simulink model "rlAutoParkingValet3D"  (R2024b)
settings: Solver=VariableStepAuto  StartTime=0.0  StopTime=inf  RelTol=1e-3  AbsTol=1e-4
InitFcn:
  | if ~doTraining
  |     setupActorVehicles(mdl,freeSpotIndex);
  | end
  | egoTargetPose = parkingLot.findGoalPose(vehiclePose,freeSpotIndex,searchDist);
StartFcn:
  | if exist("visualizer","var") && ~doTraining
  |     visualizer.resetVehicle(egoInitialPose,freeSpotIndex,doTraining);
  | end
model workspace: external: MAT-File (data not in the file)
values from neighbouring files (symbols this model uses):
  centerToRear = 1.343    [autoParkingValetParams3D.m]
  doTraining = false    [RL_Parking_And_Control.m]    (also in analisis.m; lanzarSimParalelas.m)
  egoInitialPose = [40 -55 pi/2]    [RL_Parking_And_Control.m]    (also in lanzarSimParalelas.m)
  freeSpotIndex = spotsToSimulate(i)    [RL_Parking_And_Control.m]    (also in analisis.m = 18; autoParkingValetResetFcn3D.m = 21; lanzarSimParalelas.m = 18)
  info = ParkingLotManager.getInfo()    [ParkingLotManager.m]    (also in ParkingLotVisualizer.m = this.Info; RL_Parking_And_Control.m = parkingLot.getInfo(); analisis.m = parkingLot.getInfo(); autoParkingValetResetFcn3D.m)
  K_lqr = dlqr(Ad, Bd, Q, R)    [createLQRForParking3D.m]
  maxLidarDist = 20    [autoParkingValetParams3D.m]
  parkingLot = obj.ParkingLot    [ModeSelector.m]    (also in RL_Parking_And_Control.m = ParkingLotManager; analisis.m = ParkingLotManager; lanzarSimParalelas.m = ParkingLotManager)
  pTracking = 10    [createMPCForParking3D.m]    (also in createNonLinearMPCForParking3D.m)
  searchDist = 10    [RL_Parking_And_Control.m]    (also in analisis.m; lanzarSimParalelas.m)
  speedMax = 2    [autoParkingValetParams3D.m]
  steerMax = pi/4    (= 0.785398163397)    [autoParkingValetParams3D.m]
  terrTol = deg2rad(10)    [autoParkingValetParams3D.m]
  Tf = 50    [RL_Parking_And_Control.m]    (also in analisis.m; lanzarSimParalelas.m)
  trainXBounds = info.TrainingZoneXLimits    [autoParkingValetParams3D.m]    (also in autoParkingValetResetFcn3D.m = [(info.SpotLocations(freeSpotIndex,1) - 6.8125)             )
  trainYBounds = info.TrainingZoneYLimits    [autoParkingValetParams3D.m]    (also in autoParkingValetResetFcn3D.m = [(info.SpotLocations(freeSpotIndex,2) - 9.56)              ()
  Ts = 0.1    [RL_Parking_And_Control.m]    (also in analisis.m; createMPCForParking3D.m; lanzarSimParalelas.m)
  vehiclePose = [10 -32.5 pi]    [RL_Parking_And_Control.m]    (also in analisis.m; lanzarSimParalelas.m)
  xBounds = info.XLimits    [autoParkingValetParams3D.m]
  Xref = [xRef(1:p,:);repmat(xRef(end,:),Tsteps-p,1)]    [ParkingLotManager.m]    (also in createLQRForParking3D.m = parkingLot.createReferenceTrajectory(Ts, Tf); createMPCForParking3D.m = ParkingLotManager.createReferenceTrajectory(Ts,Tf); createNonLinearMPCForParking3D.m = ParkingLotManager.createReferenceTrajectory(Ts,Tf))
  xyerrTol = 0.75    [autoParkingValetParams3D.m]
  yBounds = info.YLimits    [autoParkingValetParams3D.m]
undefined symbols (not defined in the file or in its folder): Sim3dSensor
libraries: sim3dautolib x23, simulink_extras x23, mpclib x2, rllib x1, robotmobilelib x1, sim3dphyssensorlib x1, sim3dlib x1
(part 2 of 2)

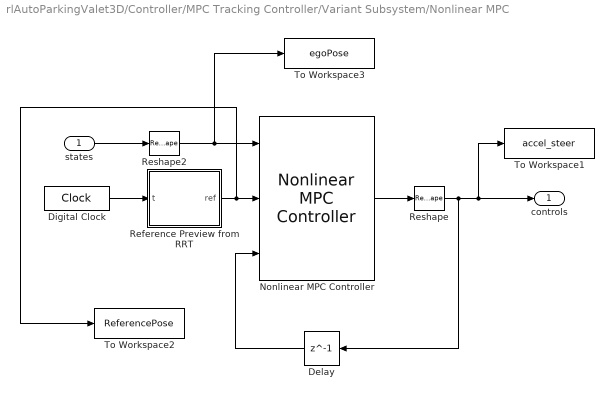
== system rlAutoParkingValet3D/Controller/MPC Tracking Controller/Variant Subsystem/Nonlinear MPC ==
  states : Inport
  Delay : Delay  DelayLength=1
  Digital Clock : DigitalClock  SampleTime=Ts
  Nonlinear MPC Controller : mpclib/Nonlinear MPC Controller  SCDEnableBlockLinearizationSpecification=on  nlmpcobj=nlobjTracking  UseObjectTs=on  UseMEX=off  md_enabled=off  mvtarget_enabled=off  param_enabled=off  cost_enabled=off  mvseq_enabled=off  stateseq_enabled=off  ovseq_enabled=off  slack_enabled=off  status_enabled=off  ov_min=off  ov_max=off  mv_min=off  mv_max=off  mvrate_min=off  mvrate_max=off  state_min=off  state_max=off  ov_weight=off  mv_weight=off  mvrate_weight=off  ecr_weight=off  nlp_initialize=off
  Reference Preview from RRT : MATLAB Function  TreatAsAtomicUnit=on
  Reshape : Reshape  OutputDimensionality=Customize  OutputDimensions=[2,1]
  Reshape2 : Reshape  OutputDimensionality=Customize  OutputDimensions=[3,1]
  To Workspace1 : ToWorkspace  VariableName=accel_steer  SaveFormat=Timeseries  SampleTime=-1
  To Workspace2 : ToWorkspace  VariableName=ReferencePose  SaveFormat=Timeseries  SampleTime=-1
  To Workspace3 : ToWorkspace  VariableName=egoPose  SaveFormat=Timeseries  SampleTime=-1
  controls : Outport
  wires:
  Nonlinear MPC Controller/1 -> Reshape/1
  Reshape/1 -> To Workspace1/1, controls/1, Delay/1
  Delay/1 -> Nonlinear MPC Controller/3
  Digital Clock/1 -> Reference Preview from RRT/1(t)
  Reference Preview from RRT/1(ref) -> To Workspace2/1, Nonlinear MPC Controller/2
  Reshape2/1 -> To Workspace3/1, Nonlinear MPC Controller/1
  states/1 -> Reshape2/1

== system rlAutoParkingValet3D/Controller/MPC Tracking Controller/Variant Subsystem/Pure Pursuit ==
  states : Inport
  Digital Clock1 : DigitalClock  SampleTime=Ts
  MATLAB Function : MATLAB Function  TreatAsAtomicUnit=on
  Reference Preview from planner : MATLAB Function  TreatAsAtomicUnit=on
  Reshape1 : Reshape  OutputDimensionality=Customize  OutputDimensions=[3,1]
  To Workspace : ToWorkspace  VariableName=egoPose  SaveFormat=Timeseries  SampleTime=-1
  To Workspace1 : ToWorkspace  VariableName=accel_steer  SaveFormat=Timeseries  SampleTime=-1
  To Workspace2 : ToWorkspace  VariableName=ReferencePose  SaveFormat=Timeseries  SampleTime=-1
  controls : Outport
  wires:
  Reference Preview from planner/1(ref) -> MATLAB Function/2(ReferencePose), To Workspace2/1  "reference"
  Reshape1/1 -> To Workspace/1, MATLAB Function/1(egoPose)
  states/1 -> Reshape1/1
  MATLAB Function/1(accel_steer) -> To Workspace1/1, controls/1
  Digital Clock1/1 -> Reference Preview from planner/1(t)

== system rlAutoParkingValet3D/Controller/MPC Tracking Controller/Variant Subsystem/Stanley ==
  states : Inport
  Digital Clock1 : DigitalClock  SampleTime=Ts
  MATLAB Function : MATLAB Function  TreatAsAtomicUnit=on
  Reference Preview from planner : MATLAB Function  TreatAsAtomicUnit=on
  Reshape1 : Reshape  OutputDimensionality=Customize  OutputDimensions=[3,1]
  To Workspace1 : ToWorkspace  VariableName=accel_steer  SaveFormat=Timeseries  SampleTime=-1
  To Workspace2 : ToWorkspace  VariableName=ReferencePose  SaveFormat=Timeseries  SampleTime=-1
  To Workspace3 : ToWorkspace  VariableName=egoPose  SaveFormat=Timeseries  SampleTime=-1
  controls : Outport
  wires:
  Reference Preview from planner/1(ref) -> To Workspace2/1, MATLAB Function/2(ReferencePose)
  Reshape1/1 -> To Workspace3/1, MATLAB Function/1(egoPose)
  states/1 -> Reshape1/1
  MATLAB Function/1(accel_steer) -> To Workspace1/1, controls/1
  Digital Clock1/1 -> Reference Preview from planner/1(t)

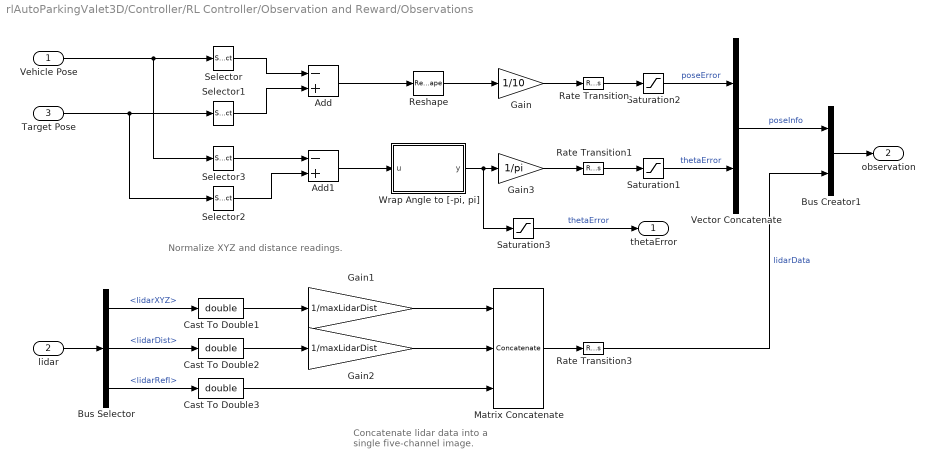
== system rlAutoParkingValet3D/Controller/RL Controller/Observation and Reward/Observations ==
  note: Concatenate lidar data into a single five-channel image.
  note: Normalize XYZ and distance readings.
  Vehicle Pose : Inport
  lidar : Inport  Port=2
  Target Pose : Inport  Port=3
  Add : Sum  Inputs=-+
  Add1 : Sum  Inputs=-+
  Bus Creator1 : BusCreator  Inputs=2  OutDataTypeStr=Bus: ObservationBus  NonVirtualBus=on
  Bus Selector : BusSelector  OutputSignals=lidarXYZ,lidarDist,lidarRefl
  Cast To Double1 : DataTypeConversion  OutDataTypeStr=double  SaturateOnIntegerOverflow=off  RndMeth=Floor
  Cast To Double2 : DataTypeConversion  OutDataTypeStr=double  SaturateOnIntegerOverflow=off  RndMeth=Floor
  Cast To Double3 : DataTypeConversion  OutDataTypeStr=double  SaturateOnIntegerOverflow=off  RndMeth=Floor
  Gain : Gain  Gain=1/10
  Gain1 : Gain  Gain=1/maxLidarDist
  Gain2 : Gain  Gain=1/maxLidarDist
  Gain3 : Gain  Gain=1/pi
  Matrix Concatenate : Concatenate  NumInputs=3  Mode=Multidimensional array  ConcatenateDimension=3
  Rate Transition : RateTransition
  Rate Transition1 : RateTransition
  Rate Transition3 : RateTransition
  Reshape : Reshape
  Saturation1 : Saturate  UpperLimit=1  LowerLimit=-1
  Saturation2 : Saturate  UpperLimit=1  LowerLimit=-1
  Saturation3 : Saturate  UpperLimit=pi  LowerLimit=-pi
  Selector : Selector  InputPortWidth=3  IndexOptions=Index vector (dialog)  Indices=1:2  OutputSizes=1
  Selector1 : Selector  InputPortWidth=3  IndexOptions=Index vector (dialog)  Indices=1:2  OutputSizes=1
  Selector2 : Selector  InputPortWidth=3  IndexOptions=Index vector (dialog)  Indices=3  OutputSizes=1
  Selector3 : Selector  InputPortWidth=3  IndexOptions=Index vector (dialog)  Indices=3  OutputSizes=1
  Vector Concatenate : Concatenate
  "Wrap Angle to [-pi, pi]" : MATLAB Function  TreatAsAtomicUnit=on
  thetaError : Outport
  observation : Outport  Port=2
  wires:
  Reshape/1 -> Gain/1
  Add/1 -> Reshape/1
  Bus Creator1/1 -> observation/1
  Selector/1 -> Add/1
  Selector1/1 -> Add/2
  "Wrap Angle to [-pi, pi]"/1(y) -> Saturation3/1, Gain3/1
  Gain/1 -> Rate Transition/1
  Gain1/1 -> Matrix Concatenate/1
  Matrix Concatenate/1 -> Rate Transition3/1
  Rate Transition/1 -> Saturation2/1
  Rate Transition1/1 -> Saturation1/1
  Vector Concatenate/1 -> Bus Creator1/1  "poseInfo"
  lidar/1 -> Bus Selector/1
  Bus Selector/1 -> Cast To Double1/1  "<lidarXYZ>"
  Bus Selector/2 -> Cast To Double2/1  "<lidarDist>"
  Bus Selector/3 -> Cast To Double3/1  "<lidarRefl>"
  Gain2/1 -> Matrix Concatenate/2
  Cast To Double1/1 -> Gain1/1
  Cast To Double2/1 -> Gain2/1
  Cast To Double3/1 -> Matrix Concatenate/3
  Target Pose/1 -> Selector2/1, Selector1/1
  Vehicle Pose/1 -> Selector3/1, Selector/1
  Selector3/1 -> Add1/1
  Add1/1 -> "Wrap Angle to [-pi, pi]"/1(u)
  Gain3/1 -> Rate Transition1/1
  Selector2/1 -> Add1/2
  Rate Transition3/1 -> Bus Creator1/2  "lidarData"
  Saturation1/1 -> Vector Concatenate/2  "thetaError"
  Saturation2/1 -> Vector Concatenate/1  "poseError"
  Saturation3/1 -> thetaError/1  "thetaError"

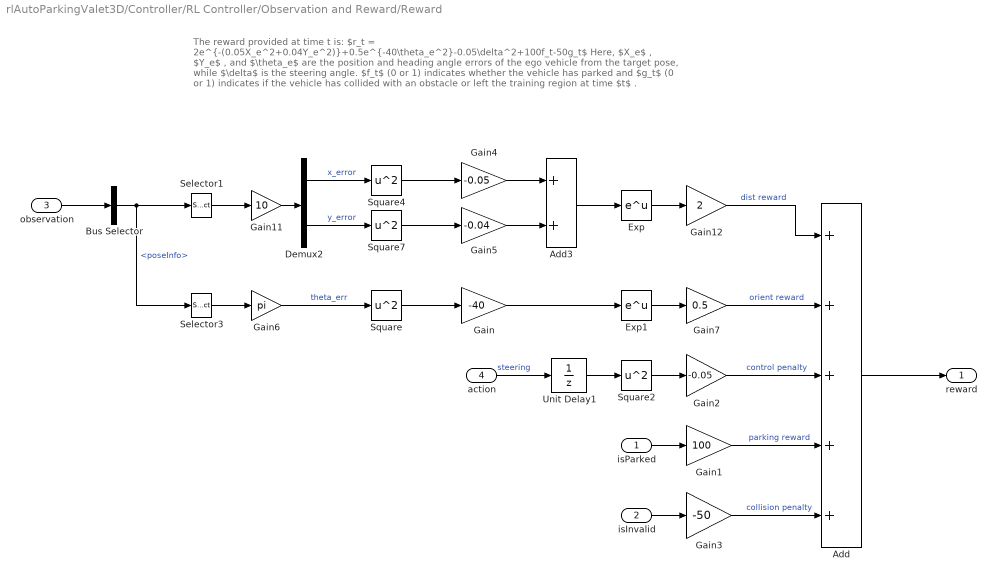
== system rlAutoParkingValet3D/Controller/RL Controller/Observation and Reward/Reward ==
  note: The reward provided at time t is:
      |
      | $r_t = 2e^{-(0.05X_e^2+0.04Y_e^2)}+0.5e^{-40\theta_e^2}-0.05\delta^2+100f_t-50g_t$
      |
      | Here, $X_e$ , $Y_e$ , and $\theta_e$ are the position and heading angle errors of the ego vehicle from the target pose, while $\delta$ is the steering angle. $f_t$ (0 or 1) indicates whether the vehicle has parked and $g_t$ (0 or 1) indicates if the vehicle has collided with an obstacle or left the training region at time $t$ .
  isParked : Inport
  isInvalid : Inport  Port=2
  observation : Inport  Port=3
  action : Inport  Port=4
  Add : Sum  Inputs=+++++
  Add3 : Sum
  Bus Selector : BusSelector  OutputSignals=poseInfo
  Demux2 : Demux  Outputs=2
  Exp : Math
  Exp1 : Math
  Gain : Gain  Gain=-40
  Gain1 : Gain  Gain=100
  Gain11 : Gain  Gain=10
  Gain12 : Gain  Gain=2
  Gain2 : Gain  Gain=-0.05
  Gain3 : Gain  Gain=-50
  Gain4 : Gain  Gain=-0.05
  Gain5 : Gain  Gain=-0.04
  Gain6 : Gain  Gain=pi
  Gain7 : Gain  Gain=0.5
  Selector1 : Selector  InputPortWidth=3  IndexOptions=Index vector (dialog)  Indices=1:2  OutputSizes=1
  Selector3 : Selector  InputPortWidth=3  IndexOptions=Index vector (dialog)  Indices=3  OutputSizes=1
  Square{,2,4,7} (4 alike) : Math  Operator=square
  Unit Delay1 : UnitDelay  SampleTime=-1  HasFrameUpgradeWarning=on
  reward : Outport
  wires:
  action/1 -> Unit Delay1/1  "steering"
  Square2/1 -> Gain2/1
  Unit Delay1/1 -> Square2/1
  Add/1 -> reward/1
  Demux2/2 -> Square7/1  "y_error"
  Square7/1 -> Gain5/1
  Square4/1 -> Gain4/1
  Add3/1 -> Exp/1
  observation/1 -> Bus Selector/1
  Demux2/1 -> Square4/1  "x_error"
  Gain4/1 -> Add3/1
  Gain5/1 -> Add3/2
  Exp/1 -> Gain12/1
  Bus Selector/1 -> Selector3/1, Selector1/1  "<poseInfo>"
  Selector3/1 -> Gain6/1
  Square/1 -> Gain/1
  Gain/1 -> Exp1/1
  Gain2/1 -> Add/3  "control penalty"
  Exp1/1 -> Gain7/1
  Gain12/1 -> Add/1  "dist reward"
  Gain7/1 -> Add/2  "orient reward"
  Gain11/1 -> Demux2/1
  isParked/1 -> Gain1/1
  Gain1/1 -> Add/4  "parking reward"
  isInvalid/1 -> Gain3/1
  Gain3/1 -> Add/5  "collision penalty"
  Selector1/1 -> Gain11/1
  Gain6/1 -> Square/1  "theta_err"

== system rlAutoParkingValet3D/Controller/RL Controller/Observation and Reward/Termination ==
  note: Terminate the episode if the vehicle successfully parks in the target spot or if it goes out-of-bounds or collides with another vehicle.
  targetPose : Inport
  Vehicle Pose : Inport  Port=2
  thetaError : Inport  Port=3
  Check Safe Area : MATLAB Function  TreatAsAtomicUnit=on  mask{LW=info.VehicleDimension, SpotId=freeSpotIndex, SpotLocations=info.SpotLocations, SpotDims=info.SpotDimension}
      mask prompts: LW "Geometry of the car [L,W]"; SpotId "Index of free parking spot"; SpotLocations "Parking lot spot locations"; SpotDims "Parking lot spot dimensions"
      mask init:
      | L = LW(1);W = LW(2);
      | spotID = SpotId;
      | spotLocations = SpotLocations;
      | spotDims = SpotDims;
  MATLAB Function : MATLAB Function  TreatAsAtomicUnit=on
  MATLAB Function1 : MATLAB Function  TreatAsAtomicUnit=on
  OR : Logic  Operator=OR  AllPortsSameDT=off  OutDataTypeStr=boolean
  isDone : Outport
  isParked : Outport  Port=2
  isInvalid : Outport  Port=3
  wires:
  OR/1 -> isDone/1
  targetPose/1 -> MATLAB Function1/2(targetpose)
  MATLAB Function1/1(y) -> OR/1, isParked/1
  MATLAB Function/1(y) -> OR/2, isInvalid/1
  Check Safe Area/1(veryCloseToObstacle) -> MATLAB Function/2(veryCloseToObstacle)
  Vehicle Pose/1 -> Check Safe Area/1(egoPose), MATLAB Function/1(vehiclePose), MATLAB Function1/1(currpose)
  thetaError/1 -> MATLAB Function1/3(thetaError)

== system rlAutoParkingValet3D/Controller/RL Controller/Observation and Reward/Translate Vehicle Origin to Centroid ==
  Rear Axle Center : Inport
  Demux1 : Demux  Outputs=3
  Mux : Mux  Inputs=3
  Translate Origin from Rear Axle to Centroid : Subsystem
  Geometric Center : Outport
  wires:
  Mux/1 -> Geometric Center/1
  Translate Origin from Rear Axle to Centroid/2(centerY) -> Mux/2
  Demux1/3 -> Mux/3, Translate Origin from Rear Axle to Centroid/3(theta)
  Demux1/2 -> Translate Origin from Rear Axle to Centroid/2(rearY)
  Rear Axle Center/1 -> Demux1/1
  Translate Origin from Rear Axle to Centroid/1(centerX) -> Mux/1
  Demux1/1 -> Translate Origin from Rear Axle to Centroid/1(rearX)

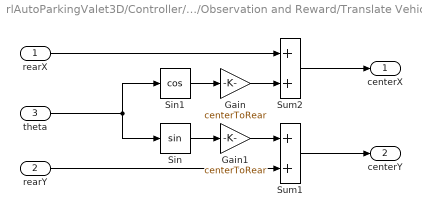
== system rlAutoParkingValet3D/Controller/RL Controller/Observation and Reward/Translate Vehicle Origin to Centroid/Translate Origin from Rear Axle to Centroid ==
  rearX : Inport
  rearY : Inport  Port=2
  theta : Inport  Port=3
  Gain : Gain  Gain=centerToRear
  Gain1 : Gain  Gain=centerToRear
  Sin : Trigonometry
  Sin1 : Trigonometry  Operator=cos
  Sum1 : Sum
  Sum2 : Sum
  centerX : Outport
  centerY : Outport  Port=2
  wires:
  Sum1/1 -> centerY/1
  rearY/1 -> Sum1/2
  theta/1 -> Sin/1, Sin1/1
  Sin/1 -> Gain1/1
  Sin1/1 -> Gain/1
  rearX/1 -> Sum2/1
  Sum2/1 -> centerX/1
  Gain/1 -> Sum2/2
  Gain1/1 -> Sum1/1

== matlab function rlAutoParkingValet3D/Controller/RL Controller/Observation and Reward/Termination/Check Safe Area ==
  data: W parameter; L parameter; egoPose input; veryCloseToObstacle output boolean; spotID parameter; spotLocations parameter; spotDims parameter
function veryCloseToObstacle = checkSafeArea(W,L,egoPose,spotID, spotLocations, spotDims)

% Calculate distances to car edges.
numPoints = 36;
angles = (0:(numPoints-1))*2*pi/numPoints;
angles = angles';
carEdges = getCarSegmentLengths(L,W,angles);

% Set X- and Y-direction tolerances.
xTol = 0.25;
yTol = 0.4;

% Get ego vehicle pose information.
X0 = egoPose(1);
Y0 = egoPose(2);
theta = egoPose(3);

% Calculate (X,Y) coordinates of vehicle edges.
X = X0 + carEdges.*cos(theta - angles);
Y = Y0 + carEdges.*sin(theta - angles);

% Check if vehicle edges violate safe zones.
veryCloseToObstacle = false;
if spotID >= 15 % Lower row of middle aisle
    if any(Y > -28)
        veryCloseToObstacle = true;
    else
        for i=1:length(carEdges)
            if (((X(i) < (spotLocations(spotID,1) - spotDims(1)/2 - xTol)) || ...
                (X(i) > (spotLocations(spotID,1) + spotDims(1)/2 + xTol)))) && ...
                (Y(i) < (spotLocations(spotID,2) + spotDims(2)/2 - yTol))
                % If any part of vehicle is outside of parking spot 
                % boundary (with tolerance), raise flag
                veryCloseToObstacle = true;
            end
        end
    end
else % Upper row of middle aisle
    if any(Y < -37)
        veryCloseToObstacle = true;
    else
        for i=1:length(carEdges)
            if (((X(i) < (spotLocations(spotID,1) - spotDims(1)/2 - xTol)) || ...
                (X(i) > (spotLocations(spotID,1) + spotDims(1)/2 + xTol)))) && ...
                (Y(i) > (spotLocations(spotID,2) - spotDims(2)/2 + yTol))
                % If any part of vehicle is outside of parking spot 
                % boundary (with tolerance), raise flag
                veryCloseToObstacle = true;
            end
        end
    end
end

== matlab function rlAutoParkingValet3D/Controller/RL Controller/Observation and Reward/Observations/Wrap Angle to [-pi, pi] ==
  data: u input; y output
function y = fcn(u)
if u < -pi
    while u < -pi
        u = u + 2*pi;
    end
elseif u > pi
    while u > pi
        u = u - 2*pi;
    end
end
y = u;

== matlab function rlAutoParkingValet3D/Controller/MPC Tracking Controller/Variant Subsystem/LQR/Reference Preview from planner ==
  data: t input; ref output; Ts parameter; Tf parameter; pTracking parameter; Xref parameter
function ref = fcn(t, Ts, Tf, pTracking, Xref)
    Tend = Tf;
    
    % Calcula los instantes de tiempo futuros (Horizonte)
    T = t + (1:pTracking) * Ts;
    T = min(T, Tend);
    
    % Genera el vector de tiempo base para la trayectoria completa
    time = Ts * (0:(size(Xref, 1) - 1));
    
    % Interpola para sacar los puntos exactos en los tiempos calculados (Matriz 10x3)
    ref = interp1(time, Xref, T);
end

== matlab function rlAutoParkingValet3D/Controller/MPC Tracking Controller/Variant Subsystem/Pure Pursuit/Reference Preview from planner ==
  data: t input; ref output; Ts parameter; Tf parameter; pTracking parameter; Xref parameter
function ref = fcn(t, Ts, Tf, pTracking, Xref)
    Tend = Tf;
    
    % Calcula los instantes de tiempo futuros (Horizonte)
    T = t + (1:pTracking) * Ts;
    T = min(T, Tend);
    
    % Genera el vector de tiempo base para la trayectoria completa
    time = Ts * (0:(size(Xref, 1) - 1));
    
    % Interpola para sacar los puntos exactos en los tiempos calculados (Matriz 10x3)
    ref = interp1(time, Xref, T);
end

== matlab function rlAutoParkingValet3D/Controller/MPC Tracking Controller/Variant Subsystem/Stanley/MATLAB Function ==
  data: egoPose input; accel_steer output; ReferencePose input; debugInfo output
function [accel_steer, debugInfo] = stanley_control(egoPose, ReferencePose)
    L = 2.8;
    v_ref = 2.5;
    dist_to_front = L / 2;   % ← antes 2.8, ahora 1.4
    
    k_stanley = 1.0;          % ← bajado de 2.0
    k_soft = 1.0;
    
    fx = egoPose(1) + dist_to_front * cos(egoPose(3));
    fy = egoPose(2) + dist_to_front * sin(egoPose(3));
    
    distancias = sqrt((ReferencePose(:,1) - fx).^2 + (ReferencePose(:,2) - fy).^2);
    [~, idx_closest] = min(distancias);
    front_ref = ReferencePose(idx_closest, :);
    
    % Mismo punto para ambos errores (Stanley puro)
    dx = fx - front_ref(1);
    dy = fy - front_ref(2);
    e_lat = (dx * sin(front_ref(3))) - (dy * cos(front_ref(3)));
    
    theta_e = front_ref(3) - egoPose(3);
    theta_e = atan2(sin(theta_e), cos(theta_e));
    
    delta = theta_e + atan((k_stanley * e_lat) / (v_ref + k_soft));
    
    u = [v_ref; max(-pi/4, min(pi/4, delta))];
    accel_steer = u;
    debugInfo = e_lat;
end

== matlab function rlAutoParkingValet3D/Controller/MPC Tracking Controller/Variant Subsystem/Stanley/Reference Preview from planner ==
  data: t input; ref output; Ts parameter; Tf parameter; pTracking parameter; Xref parameter
function ref = fcn(t, Ts, Tf, pTracking, Xref)
    Tend = Tf;
    
    % Calcula los instantes de tiempo futuros (Horizonte)
    T = t + (1:pTracking) * Ts;
    T = min(T, Tend);
    
    % Genera el vector de tiempo base para la trayectoria completa
    time = Ts * (0:(size(Xref, 1) - 1));
    
    % Interpola para sacar los puntos exactos en los tiempos calculados (Matriz 10x3)
    ref = interp1(time, Xref, T);
end

== matlab function rlAutoParkingValet3D/Controller/MPC Tracking Controller/Variant Subsystem/Nonlinear MPC/Reference Preview from RRT ==
  data: t input; ref output; Ts parameter; Tf parameter; pTracking parameter; Xref parameter
function ref = fcn(t,Ts,Tf,pTracking,Xref)
Tend = Tf;
T = t+(1:pTracking)*Ts;
T = min(T,Tend);
time = Ts*(1:length(Xref));
ref = interp1(time,Xref,T);

== matlab function rlAutoParkingValet3D/Controller/RL Controller/Observation and Reward/Termination/MATLAB Function ==
  data: vehiclePose input; veryCloseToObstacle input; y output; xBounds parameter; yBounds parameter; trainXBounds parameter; trainYBounds parameter; doTraining parameter; egoInitialPose parameter
function y = isOutOfBounds(vehiclePose, veryCloseToObstacle, xBounds, yBounds, trainXBounds, trainYBounds, doTraining, egoInitialPose)

if doTraining
    xlims = trainXBounds;
    ylims = trainYBounds;
else
    xlims = xBounds;
    ylims = yBounds;
end

% get coordinates of four corners
xc = vehiclePose(1);
yc = vehiclePose(2);
t  = vehiclePose(3);

% threshold
tol = 0.1;

% Check if true positions are out of bounds
xOutOfBounds = xc <= xlims(1) + tol || xc >= xlims(2) - tol;
yOutOfBounds = yc <= ylims(1) + tol || yc >= ylims(2) - tol;

% check if lidar reading is less than threshold value
% veryCloseToObstacle = lidarMinDist <= lidarTol;

goingInCircles = false;
if doTraining
    % goingInCircles = (t > 3*pi) || (t < -pi);
    goingInCircles = (t > egoInitialPose(3) + 2*pi) || (t < egoInitialPose(3) - 2*pi);
end

y = xOutOfBounds || yOutOfBounds || veryCloseToObstacle || goingInCircles;

== matlab function rlAutoParkingValet3D/Controller/MPC Tracking Controller/Variant Subsystem/Pure Pursuit/MATLAB Function ==
  data: egoPose input; accel_steer output; ReferencePose input; debugInfo output
function [accel_steer, debugInfo] = pure_pursuit_control(egoPose, ReferencePose)
    % --- 1. PARÁMETROS BASE ---
    L = 2.8;
    v_ref = 2.0;

    % --- 2. TRASLACIÓN AL EJE TRASERO ---
    dist_to_rear = L / 2;
    rear_x = egoPose(1) - dist_to_rear * cos(egoPose(3));
    rear_y = egoPose(2) - dist_to_rear * sin(egoPose(3));

    % --- 3. PUNTO MÁS CERCANO ---
    distancias = sqrt((ReferencePose(:,1) - rear_x).^2 + ...
                      (ReferencePose(:,2) - rear_y).^2);
    [~, idx_closest] = min(distancias);

    % --- 4. CURVATURA ANTICIPADA (ventana solo hacia adelante) ---
    % Medimos el cambio de heading entre dos puntos futuros, no incluimos
    % nada del pasado. Esto da anticipación real al inicio de la curva.
    N = size(ReferencePose,1);
    idx_near   = min(idx_closest + 5,  N);
    idx_mid    = min(idx_closest + 15, N);
    idx_far    = min(idx_closest + 30, N);

    % Curvatura entre el punto cercano-futuro y el medio-futuro
    diff_1 = ReferencePose(idx_mid, 3) - ReferencePose(idx_near, 3);
    diff_1 = abs(atan2(sin(diff_1), cos(diff_1)));

    % Curvatura entre el punto medio-futuro y el lejano-futuro
    diff_2 = ReferencePose(idx_far, 3) - ReferencePose(idx_mid, 3);
    diff_2 = abs(atan2(sin(diff_2), cos(diff_2)));

    % Tomamos la máxima: si CUALQUIERA de las dos zonas tiene curva,
    % activamos modo curva. Esto anticipa antes y mantiene Ld bajo
    % durante toda la curva (entrada y salida).
    diff_path = max(diff_1, diff_2);

    % --- 5. Ld ADAPTATIVO CON TRANSICIÓN NO LINEAL ---
    % Usamos sqrt() para que Ld baje rápido en cuanto hay un poco de
    % curvatura, en lugar de hacerlo linealmente.
    curvatura_norm = min(1.0, diff_path / 0.30);
    curvatura_norm = sqrt(curvatura_norm);   % transición agresiva

    Ld_recta = 14.0;
    Ld_curva = 1.5;
    Ld = Ld_recta - curvatura_norm * (Ld_recta - Ld_curva);

    % Suelo mínimo
    Ld = max(Ld, 3.0);

    % --- 6. SELECCIÓN DEL PUNTO OBJETIVO ---
    target_idx = N;
    for i = idx_closest:N
        if distancias(i) >= Ld
            target_idx = i;
            break;
        end
    end
    target_pt = ReferencePose(target_idx, :);

    % --- 7. ALPHA ---
    dx = target_pt(1) - rear_x;
    dy = target_pt(2) - rear_y;
    alpha = atan2(dy, dx) - egoPose(3);
    alpha = atan2(sin(alpha), cos(alpha));

    % --- 8. LEY DE PURE PURSUIT ---
    delta = atan2(2 * L * sin(alpha), Ld);

    % --- 9. SATURACIÓN Y SALIDA ---
    u = [v_ref; max(-1, min(1, delta))];
    accel_steer = u;
    debugInfo = Ld;
end

== matlab function rlAutoParkingValet3D/Vehicle Dynamics and Sensing/Unreal Engine Visualization and Sensing/MATLAB Function ==
  data: pose input; steer input; isParking input; doTraining input
function plot2DVehicle(pose,steer,isParking,doTraining)
    coder.extrinsic('plotVehicle');
    plotVehicle(pose,steer,isParking,doTraining);
end

== matlab function rlAutoParkingValet3D/Controller/RL Controller/Observation and Reward/Termination/MATLAB Function1 ==
  data: currpose input; y output; targetpose input; xyerrTol parameter; terrTol parameter; thetaError input
function y = isParked(currpose,targetpose, xyerrTol, terrTol, thetaError)

x = currpose(1);
y = currpose(2);
xg = targetpose(1);
yg = targetpose(2);
xyerr = sqrt((x-xg)^2+(y-yg)^2);
y = 0;
if xyerr < xyerrTol && abs(thetaError) < terrTol
    y = 1;
end

== matlab function rlAutoParkingValet3D/Controller/MPC Tracking Controller/Variant Subsystem/LQR/MATLAB Function ==
  data: egoPose input; accel_steer output; ReferencePose input; K_lqr input; debugInfo output
function [accel_steer, debugInfo] = lqr_control(egoPose, ReferencePose, K_lqr)
    v_ref = 2.5; 
    u_nom = [v_ref; 0]; 
    
    current_ref = ReferencePose(1, :);
    
    % 1. Calcular el error global
    dx = egoPose(1) - current_ref(1);
    dy = egoPose(2) - current_ref(2);
    dtheta = egoPose(3) - current_ref(3);
    
    % Normalizar el ángulo entre -pi y pi
    dtheta = atan2(sin(dtheta), cos(dtheta));
    
    % 2. ROTAR EL ERROR AL MARCO LOCAL (Transformación fundamental)
    % Usamos el ángulo de la referencia para saber qué es "adelante" y qué es "lados"
    theta_ref = current_ref(3);
    e_lon =  dx * cos(theta_ref) + dy * sin(theta_ref);
    e_lat = -dx * sin(theta_ref) + dy * cos(theta_ref);
    
    % Agrupamos el nuevo error local
    error_local = [e_lon; e_lat; dtheta];
    
    % 3. Aplicar LQR sobre el error local
    u = u_nom - (K_lqr * error_local);
    
    % 4. Saturación (Límites físicos)
    u(1) = max(-5, min(5, u(1)));         
    u(2) = max(-pi/4, min(pi/4, u(2)));   
    
    accel_steer = u;
    debugInfo = 0; 
end

== matlab function rlAutoParkingValet3D/Controller/MPC Tracking Controller/Variant Subsystem/Adaptive MPC/Plant Model Generator ==
  settings: updateMethod=DISCRETE  sampleTime=Ts
  data: x input size=[3,1]; u input size=[2,1]; A output; B output; C output; D output; U output size=[2,1]; Y output size=[3,1]; X output size=[3,1]; DX output size=[3,1]; Ts parameter
function [A,B,C,D,U,Y,X,DX] = fcn(x,u,Ts)

[A,B,C,D,U,Y,X,DX] = vehicleStateJacobianFcnDT(Ts,x,u);

== matlab function rlAutoParkingValet3D/Controller/MPC Tracking Controller/Variant Subsystem/Adaptive MPC/Reference Preview from planner ==
  data: t input; ref output; Ts parameter; Tf parameter; pTracking parameter; Xref parameter
function ref = fcn(t,Ts,Tf,pTracking,Xref)
Tend = Tf;
T = t+(1:pTracking)*Ts;
T = min(T,Tend);
time = Ts*(1:length(Xref*1.2));
ref = interp1(time,Xref,T);
